simulink model "CRH2forBenchmark_Copy"  (R2014a)
settings: Solver=ode3  StartTime=0.0  StopTime=1  FixedStep=1e-5  RelTol=1e-3
PostLoadFcn:
  | , if any(exist('dsrtsu_mdlpostloadfcn', 'file') == [2, 3, 6]), try dsrtsu_mdlpostloadfcn('Execute', bdroot); catch fprintf('Error in PostLoadFcn (dsrtsu_mdlpostloadfcn) for model "%s":\n %s\n', bdroot, lasterr); end, end,
values from neighbouring files (symbols this model uses):
  Cd = 0.016    [CRH2forBenchmark.mat]
  Lm = 0.032848    [CRH2forBenchmark.mat]
  Ln = 0.002    [CRH2forBenchmark.mat]
  Lr = 0.034142    [CRH2forBenchmark.mat]
  Ls = 0.0342654    [CRH2forBenchmark.mat]
  np = 2    [CRH2forBenchmark.mat]
  Rd = 6000    [CRH2forBenchmark.mat]
  Rn = 0.2    [CRH2forBenchmark.mat]
  Rr = 0.146    [CRH2forBenchmark.mat]
  Rs = 0.144    [CRH2forBenchmark.mat]
  ts = 1e-05    [CRH2forBenchmark.mat]
undefined symbols (not defined in the file): J, KIM, KIT, KPM, KPT, phir, Ts, Vge
libraries: simulink x20
(part 5 of 5)

== system CRH2forBenchmark_Copy/ConverterN/Rectifier/RecSubN/SBN/__InputSSForSFun__ ==
  Tb1 : Inport
  Tb2 : Inport  Port=2
  Tb3 : Inport  Port=3
  Tb4 : Inport  Port=4
  In : Inport  Port=5
  __UniqueOutportName__1__ : Outport
  __UniqueOutportName__2__ : Outport  Port=2
  __UniqueOutportName__3__ : Outport  Port=3
  __UniqueOutportName__4__ : Outport  Port=4
  __UniqueOutportName__5__ : Outport  Port=5
  wires:
  Tb1/1 -> __UniqueOutportName__1__/1
  Tb2/1 -> __UniqueOutportName__2__/1
  Tb3/1 -> __UniqueOutportName__3__/1
  Tb4/1 -> __UniqueOutportName__4__/1
  In/1 -> __UniqueOutportName__5__/1

== system CRH2forBenchmark_Copy/ConverterN/Rectifier/RecSubN/SBN/__OutputSSForSFun__ ==
  __UniqueInportName__1__ : Inport
  SB : Outport
  wires:
  __UniqueInportName__1__/1 -> SB/1

== system CRH2forBenchmark_Copy/Benchmark/MFI1/MFI1/MFI /MFI1/__InputSSForSFun__ ==
  Nomal : Inport
  Outside Signal1 : Inport  Port=2
  __UniqueOutportName__1__ : Outport
  __UniqueOutportName__2__ : Outport  Port=2
  __UniqueOutportName__3__ : Outport  Port=3
  wires:
  [NoiseMFI1] -> __UniqueOutportName__3__/1
  Outside Signal1/1 -> __UniqueOutportName__2__/1
  Nomal/1 -> __UniqueOutportName__1__/1

== system CRH2forBenchmark_Copy/Benchmark/MFI1/MFI1/MFI /MFI1/__OutputSSForSFun__ ==
  __UniqueInportName__1__ : Inport
  Out : Outport
  wires:
  __UniqueInportName__1__/1 -> Out/1

== system CRH2forBenchmark_Copy/Benchmark/MFI1/MFI2/MFI /MFI1/__InputSSForSFun__ ==
  Nomal : Inport
  Outside Signal1 : Inport  Port=2
  __UniqueOutportName__1__ : Outport
  __UniqueOutportName__2__ : Outport  Port=2
  __UniqueOutportName__3__ : Outport  Port=3
  wires:
  Nomal/1 -> __UniqueOutportName__1__/1
  Outside Signal1/1 -> __UniqueOutportName__2__/1
  [NoiseMFI2] -> __UniqueOutportName__3__/1

== system CRH2forBenchmark_Copy/Benchmark/MFI1/MFI2/MFI /MFI1/__OutputSSForSFun__ ==
  __UniqueInportName__1__ : Inport
  Out : Outport
  wires:
  __UniqueInportName__1__/1 -> Out/1

== system CRH2forBenchmark_Copy/Benchmark/MFI1/MFI3/MFI /MFI1/__InputSSForSFun__ ==
  Nomal : Inport
  Outside Signal1 : Inport  Port=2
  __UniqueOutportName__1__ : Outport
  __UniqueOutportName__2__ : Outport  Port=2
  __UniqueOutportName__3__ : Outport  Port=3
  wires:
  [NoiseMFI3] -> __UniqueOutportName__3__/1
  Outside Signal1/1 -> __UniqueOutportName__2__/1
  Nomal/1 -> __UniqueOutportName__1__/1

== system CRH2forBenchmark_Copy/Benchmark/MFI1/MFI3/MFI /MFI1/__OutputSSForSFun__ ==
  __UniqueInportName__1__ : Inport
  Out : Outport
  wires:
  __UniqueInportName__1__/1 -> Out/1

== system CRH2forBenchmark_Copy/Benchmark/MFI1/MFI4/MFI /MFI1/__InputSSForSFun__ ==
  Nomal : Inport
  Outside Signal1 : Inport  Port=2
  __UniqueOutportName__1__ : Outport
  __UniqueOutportName__2__ : Outport  Port=2
  __UniqueOutportName__3__ : Outport  Port=3
  wires:
  [NoiseMFI4] -> __UniqueOutportName__3__/1
  Outside Signal1/1 -> __UniqueOutportName__2__/1
  Nomal/1 -> __UniqueOutportName__1__/1

== system CRH2forBenchmark_Copy/Benchmark/MFI1/MFI4/MFI /MFI1/__OutputSSForSFun__ ==
  __UniqueInportName__1__ : Inport
  Out : Outport
  wires:
  __UniqueInportName__1__/1 -> Out/1

== system CRH2forBenchmark_Copy/Benchmark/MFI1/MFI5/MFI /MFI1/__InputSSForSFun__ ==
  Nomal : Inport
  Outside Signal1 : Inport  Port=2
  __UniqueOutportName__1__ : Outport
  __UniqueOutportName__2__ : Outport  Port=2
  __UniqueOutportName__3__ : Outport  Port=3
  wires:
  Nomal/1 -> __UniqueOutportName__1__/1
  Outside Signal1/1 -> __UniqueOutportName__2__/1
  [NoiseMFI5] -> __UniqueOutportName__3__/1

== system CRH2forBenchmark_Copy/Benchmark/MFI1/MFI5/MFI /MFI1/__OutputSSForSFun__ ==
  __UniqueInportName__1__ : Inport
  Out : Outport
  wires:
  __UniqueInportName__1__/1 -> Out/1

== system CRH2forBenchmark_Copy/Benchmark/MFI1/MFI6/MFI /MFI1/__InputSSForSFun__ ==
  Nomal : Inport
  Outside Signal1 : Inport  Port=2
  __UniqueOutportName__1__ : Outport
  __UniqueOutportName__2__ : Outport  Port=2
  __UniqueOutportName__3__ : Outport  Port=3
  wires:
  Nomal/1 -> __UniqueOutportName__1__/1
  Outside Signal1/1 -> __UniqueOutportName__2__/1
  [NoiseMFI6] -> __UniqueOutportName__3__/1

== system CRH2forBenchmark_Copy/Benchmark/MFI1/MFI6/MFI /MFI1/__OutputSSForSFun__ ==
  __UniqueInportName__1__ : Inport
  Out : Outport
  wires:
  __UniqueInportName__1__/1 -> Out/1

== matlab function CRH2forBenchmark_Copy/Benchmark/TFI1/TFI1Sub/Logic Operation/MATLAB Function ==
  data: x input; y output; Num input
function y   = fa(x,Num)
%FA Summary of this function goes here
%   Detailed explanation goes here
if x<0
    x=-x;
    bin = dec2bin(x,16);
    randdata = Num;
    bin(randdata);
    if bin(randdata)=='1'
        bin(randdata) = '0';
    else
        bin(randdata) = '1';
    end
%     bin;
    y = bin2dec(bin);
    y=-y;
 else
    bin = dec2bin(x,16);
    randdata = Num;
    bin(randdata);
    if bin(randdata)=='1'
        bin(randdata) = '0';
    else
        bin(randdata) = '1';
    end
%     bin;
    y = bin2dec(bin);

end
